simulink model "LinPendLQ"  (R2023a)
settings: Solver=ode45  StartTime=0.0  StopTime=Tmax  RelTol=1e-6  EnableMultiTasking=on
values from neighbouring files (symbols this model uses):
  a = g / L    (= 32.6666666667)    [mLinPendLQR.m]
  b = k / m    (= 0.0333333333333)    [mLinPendLQR.m]
  c = 1 / (m * L ^ 2)    (= 37.037037037)    [mLinPendLQR.m]
  h = 0.1    [mLinPendLQR.m]
  umax = 0.34    [mLinPendLQR.m]
undefined symbols (not defined in the file or in its folder): KLQ
settings Model: Creator=jomle  LastModifiedBy=ruipe
settings SolverCC: AlgebraicLoopSolver=TrustRegion
settings DataIOCC: LimitDataPoints=on  SaveFormat=Array  ReturnWorkspaceOutputs=off
settings OptimizationCC: LifeSpan=inf
settings DebuggingCC: UnconnectedInputMsg=warning  UnconnectedOutputMsg=warning  UnconnectedLineMsg=warning  SFUnexpectedBacktrackingDiag=warning  SFNoUnconditionalDefaultTransitionDiag=warning  SFExecutionAtInitializationDiag=none  ArithmeticOperatorsInVariantConditions=warning
settings HardwareCC: ProdBitPerPointer=32  ProdBitPerSizeT=32  ProdBitPerPtrDiffT=32  ProdLargestAtomicFloat=None  ProdIntDivRoundTo=Undefined  ProdEndianess=Unspecified  ProdWordSize=32  ProdHWDeviceType=32-bit Generic
settings ModelReferenceCC: PropagateSignalLabelsOutOfModel=off
settings SFSimCC: SimUseLocalCustomCode=off  CustomCodeUndefinedFunction=UseInterfaceOnly
settings RTWCC: RTWUseLocalCustomCode=off
settings CodeAppCC: StateflowObjectComments=on
settings GRTTargetCC: TargetLangStandard=C89/C90 (ANSI)
settings ConfigComp: CovMetricSettings=dw  CovSaveCumulativeToWorkspaceVar=on  CovSaveSingleToWorkspaceVar=on  CovExternalEMLEnable=off

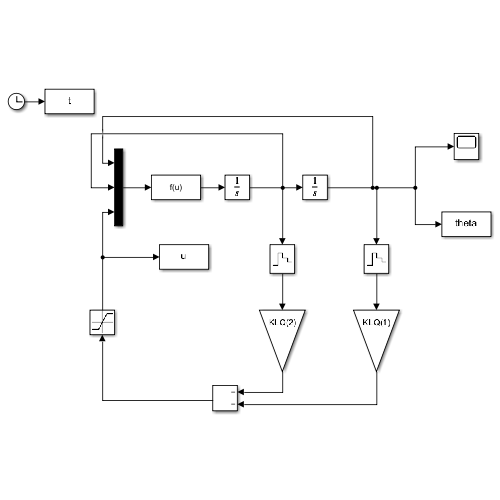
[thumbnail: Simulink's stored preview of the top-level diagram]
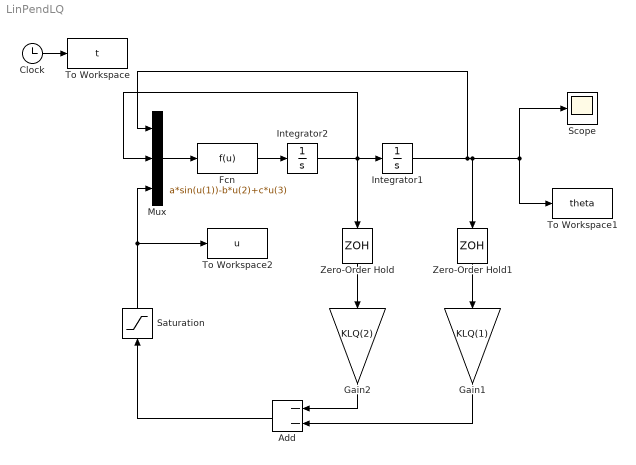
== system LinPendLQ ==
  Add : Sum  Inputs=--
  Clock : Clock
  Fcn : Fcn  Expr=a*sin(u(1))-b*u(2)+c*u(3)
  Gain1 : Gain  Gain=KLQ(1)
  Gain2 : Gain  Gain=KLQ(2)
  Integrator1 : Integrator  InitialCondition=pi/8
  Integrator2 : Integrator
  Mux : Mux  Inputs=3
  Saturation : Saturate  UpperLimit=umax  LowerLimit=-umax
  Scope : Scope
  To Workspace : ToWorkspace  VariableName=t  SampleTime=-1
  To Workspace1 : ToWorkspace  VariableName=theta  SampleTime=-1
  To Workspace2 : ToWorkspace  VariableName=u  SaveFormat=Structure With Time  SampleTime=-1
  Zero-Order Hold : ZeroOrderHold  SampleTime=h
  Zero-Order Hold1 : ZeroOrderHold  SampleTime=h
  wires:
  Integrator2/1 -> Mux/2, Zero-Order Hold/1, Integrator1/1
  Integrator1/1 -> To Workspace1/1, Scope/1, Zero-Order Hold1/1, Mux/1
  Mux/1 -> Fcn/1
  Fcn/1 -> Integrator2/1
  Gain2/1 -> Add/1
  Gain1/1 -> Add/2
  Add/1 -> Saturation/1
  Clock/1 -> To Workspace/1
  Zero-Order Hold/1 -> Gain2/1
  Zero-Order Hold1/1 -> Gain1/1
  Saturation/1 -> To Workspace2/1, Mux/3
